simulink model "ORC_test_simu_feedback"  (R2018a)
settings: Solver=VariableStepAuto  StartTime=0.0  StopTime=9  RelTol=1e-4
undefined symbols (not defined in the file or in its folder): handle_sink, handle_source, handle_wf, pe, sigbuilder_block
libraries: pe_lib x1
(part 1 of 3)
settings Model: Creator=njgreen3  LastModifiedBy=njgreen3
settings SolverCC: AlgebraicLoopSolver=LineSearch
settings DebuggingCC: ParameterOverflowMsg=warning

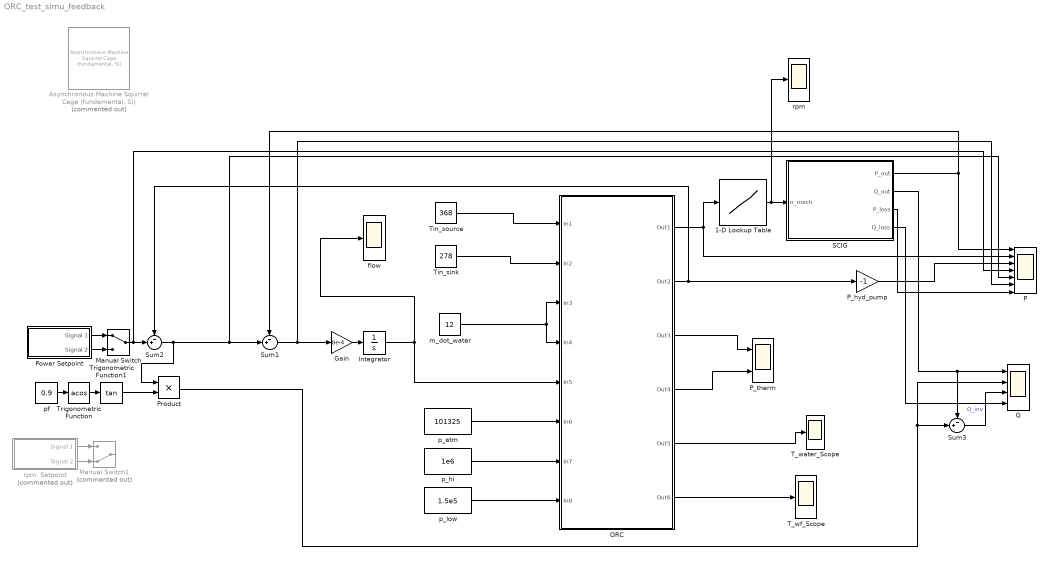
== system ORC_test_simu_feedback ==
  1-D Lookup Table : Lookup_n-D  NumberOfTableDimensions=1  BreakpointsForDimension1="-1/3*[166663.989372846\t163937.628261044\t155852.617467788\t140628.948970298\t116654.771019611\t83123.6124212207\t40806.0621676137\t-7481.19463142690\t-57239.4174183274\t-103560.341265182\t-142633.126036591\t-172599.754334336\t-193461.262910890\t-206409.980979167\t-213110.460435838\t-215209.127126632]"  Table="[834.591559026165\t844.140855611678\t853.690152197192\t863.239448782706\t872.788745368220\t882.338041953733\t891.887338539247\t901.436635124761\t910.985931710274\t920.535228295788\t930.084524881302\t939.633821466816\t949.183118052329\t958.732414637843\t968.281711223357\t977.831007808871]"  ExtrapMethod=Clip  DiagnosticForOutOfRangeInput=Error  InternalRulePriority=Speed  RndMeth=Simplest  InputSameDT=on
  "Asynchronous Machine Squirrel Cage (fundamental, SI)" : pe_lib/Machines/Asynchronous Machine (Squirrel Cage)/Asynchronous Machine Squirrel Cage (fundamental, SI)  Commented=on  SRated=40e3 V*A  VRated=220 V  FRated=60 Hz  nPolePairs=4  zero_sequence=pe.enum.park.zerosequence.include  Rs=0.018 Ohm  Xls=0.32 Ohm  Rrd=0.03 Ohm  Xlrd=0.05 Ohm  Xm=18 Ohm  X0=0.9 Ohm  connection_option=int32(pe.Connection.delta)  base_psi=nan Wb  angular_position_specify=off  angular_position_priority=None  angular_position=0 deg  angular_position_nominal_specify=off  angular_position_nominal_unit=deg  angular_position_nominal_value=1  psids_specify=off  psids_priority=None  psids=0 Wb  psids_nominal_specify=off  psids_nominal_unit=Wb  psids_nominal_value=1  psiqs_specify=off  psiqs_priority=None  psiqs=0 Wb  psiqs_nominal_specify=off  psiqs_nominal_unit=Wb  psiqs_nominal_value=1  psidr_specify=off  psidr_priority=None  psidr=0 Wb  psidr_nominal_specify=off  psidr_nominal_unit=Wb  psidr_nominal_value=1  psiqr_specify=off  psiqr_priority=None  psiqr=0 Wb  psiqr_nominal_specify=off  psiqr_nominal_unit=Wb  psiqr_nominal_value=1
      settings: SourceProductName=Simscape Power Systems  SourceProductBaseCode=PS
  Gain : Gain  Gain=8e-4
  Integrator : Integrator  InitialCondition=3  UpperSaturationLimit=8  LowerSaturationLimit=0
  Manual Switch : ManualSwitch
  Manual Switch1 : ManualSwitch  Commented=on  CurrentSetting=0
  ORC : Subsystem
  P : Scope  NumInputPorts=7
  P_hyd_pump : Gain  Gain=-1
  P_therm : Scope  NumInputPorts=2
  Power Setpoint : Subsystem  Tag=STV Subsys  LoadFcn=sigbuilder_block('load');  StartFcn=sigbuilder_block('start');  StopFcn=sigbuilder_block('stop');  ClipboardFcn=sigbuilder_block('clipboard');  mask(Sigbuilder block){tuvar=[0:10]}
      mask help: Simulink:masks:SigbuilderBlock_MD
      mask init:
      | if ~strcmp(get_param(bdroot(gcbh),'SimulationStatus'),'stopped') tuvar = sigbuilder_block('maskInit'); end
      settings: CopyFcn=sigbuilder_block('copy');  DeleteFcn=sigbuilder_block('delete');  ModelCloseFcn=sigbuilder_block('modelClose');  PreSaveFcn=sigbuilder_block('preSave');  PauseFcn=sigbuilder_block('pause');  ContinueFcn=sigbuilder_block('continue');  NameChangeFcn=sigbuilder_block('namechange');  OpenFcn=sigbuilder_block('open',[440.25 156.75 544.5 355.5 ]);  CloseFcn=sigbuilder_block('close');
      mask Display: plot(0, 0, 100, 100,[2, 2, 32, 32, 2], [68, 8, 8, 68, 68],[32, 2], [38, 38], [32, 19, 2],[53, 60, 44], [32, 17, 17, 2],[16, 16, 31, 31]);txt = getActiveGroup(gcbh);text(2, 100, txt,'verticalAlignment', 'top');
  Product : Product
  Q : Scope  NumInputPorts=4
  SCIG : MATLAB Function  TreatAsAtomicUnit=on  mask{Vll=220, f_synch=60, poles=4, R1=0.018, X1=0.32, R2=0.03, X2=0.05, Rm=5000, Xm=18, Rx=.003, Xx=12, K_b=0, K_w=0}
      mask prompts: Vll "Line Voltage (V)"; f_synch "Frequency (Hz)"; poles "Pole Pairs"; R1 "Stator Resistance, Rs"; X1 "Stator Reactance, Xs"; R2 "Referred Rotor Resistance, Rr'"; X2 "Reffered Rotor Reactance, Xr'"; Rm "Magnetizing Resistance of Core, Rm"; Xm "Magnetizing Reactance of Core, Xm"; Rx "Equivalent Series Resistance (ESR) of excitationm, Rx"; Xx "Excitation capacitance, Xx"; K_b "Coefficient of Bearing Friction, Kb"; K_w "Coefficient of Windage Friction, Kw"
  Sum1 : Sum  Inputs=-+|
  Sum2 : Sum  Inputs=-+|
  Sum3 : Sum  Inputs=-+|
  T_water_Scope : Scope
  T_wf_Scope : Scope
  Tin_sink : Constant  Value=278
  Tin_source : Constant  Value=368
  Trigonometric Function : Trigonometry  Operator=acos
  Trigonometric Function1 : Trigonometry  Operator=tan
  flow : Scope
  m_dot_water : Constant  Value=12
  p_atm : Constant  Value=101325
  p_hi : Constant  Value=1e6
  p_low : Constant  Value=1.5e5
  pf : Constant  Value=0.9
  rpm : Scope
  rpm  Setpoint : Subsystem  Tag=STV Subsys  Commented=on  LoadFcn=sigbuilder_block('load');  StartFcn=sigbuilder_block('start');  StopFcn=sigbuilder_block('stop');  ClipboardFcn=sigbuilder_block('clipboard');  mask(Sigbuilder block){tuvar=[0:10]}
      mask help: Simulink:masks:SigbuilderBlock_MD
      mask init:
      | if ~strcmp(get_param(bdroot(gcbh),'SimulationStatus'),'stopped') tuvar = sigbuilder_block('maskInit'); end
      settings: CopyFcn=sigbuilder_block('copy');  DeleteFcn=sigbuilder_block('delete');  ModelCloseFcn=sigbuilder_block('modelClose');  PreSaveFcn=sigbuilder_block('preSave');  PauseFcn=sigbuilder_block('pause');  ContinueFcn=sigbuilder_block('continue');  NameChangeFcn=sigbuilder_block('namechange');  OpenFcn=sigbuilder_block('open',[674.25 225 550.5 399.75 ]);  CloseFcn=sigbuilder_block('close');
      mask Display: plot(0, 0, 100, 100,[2, 2, 32, 32, 2], [68, 8, 8, 68, 68],[32, 2], [38, 38], [32, 19, 2],[53, 60, 44], [32, 17, 17, 2],[16, 16, 31, 31]);txt = getActiveGroup(gcbh);text(2, 100, txt,'verticalAlignment', 'top');
  wires:
  Tin_source/1 -> ORC/1(In1)
  m_dot_water/1 -> ORC/3(In3), ORC/4(In4)
  p_atm/1 -> ORC/6(In6)
  p_hi/1 -> ORC/7(In7)
  p_low/1 -> ORC/8(In8)
  ORC/3(Out3) -> P_therm/1
  ORC/4(Out4) -> P_therm/2
  ORC/5(Out5) -> T_water_Scope/1
  ORC/6(Out6) -> T_wf_Scope/1
  Tin_sink/1 -> ORC/2(In2)
  Gain/1 -> Integrator/1
  Power Setpoint/1(Signal 1) -> Manual Switch/1
  Power Setpoint/2(Signal 2) -> Manual Switch/2
  Manual Switch/1 -> P/4, Sum2/2
  pf/1 -> Trigonometric Function/1
  Trigonometric Function/1 -> Trigonometric Function1/1
  Trigonometric Function1/1 -> Product/2
  Product/1 -> Sum3/2, Q/2
  Sum2/1 -> P/5, Sum1/2, Product/1
  rpm  Setpoint/1(Signal 1) -> Manual Switch1/1
  rpm  Setpoint/2(Signal 2) -> Manual Switch1/2
  Integrator/1 -> ORC/5(In5), flow/1
  ORC/1(Out1) -> P/2, 1-D Lookup Table/1
  1-D Lookup Table/1 -> rpm/1, SCIG/1(n_mech)
  ORC/2(Out2) -> Sum2/1, P_hyd_pump/1
  SCIG/1(P_out) -> Sum1/1, P/1
  P_hyd_pump/1 -> P/3
  Sum1/1 -> P/6, Gain/1
  SCIG/2(Q_out) -> Sum3/1, Q/1
  Sum3/1 -> Q/3  "Q_inv"
  SCIG/4(Q_loss) -> Q/4
  SCIG/3(P_loss) -> P/7

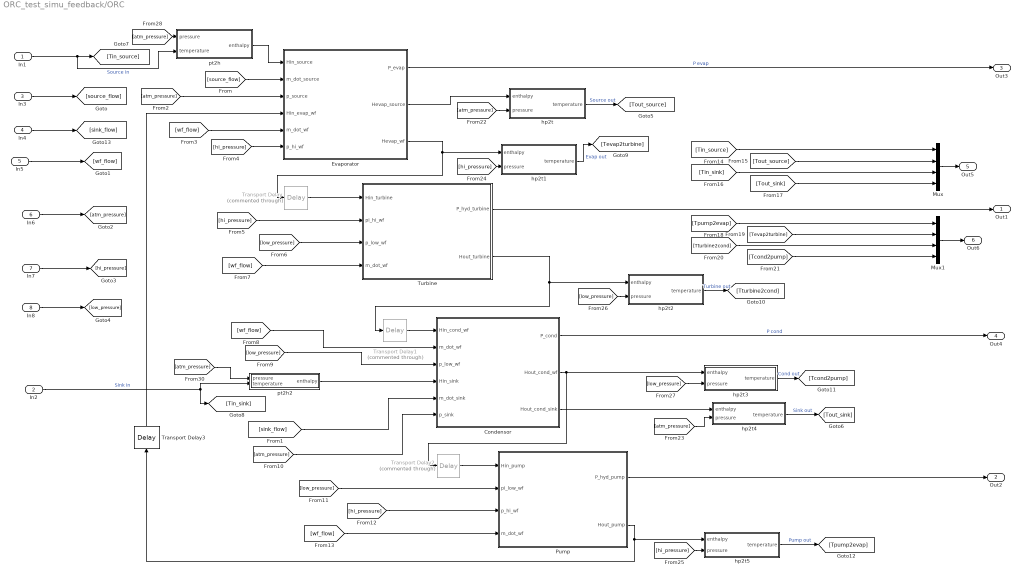
== system ORC_test_simu_feedback/ORC ==
  In1 : Inport
  In2 : Inport  Port=2
  In3 : Inport  Port=3
  In4 : Inport  Port=4
  In5 : Inport  Port=5
  In6 : Inport  Port=6
  In7 : Inport  Port=7
  In8 : Inport  Port=8
  Condensor : Subsystem
  Evaporator : Subsystem
  Mux : Mux
  Mux1 : Mux
  Pump : Subsystem
  Transport Delay : TransportDelay  Commented=through  DelayTime=.01  InitialOutput=2.3e+05
  Transport Delay1 : TransportDelay  Commented=through  DelayTime=.01  InitialOutput=2.3e+05
  Transport Delay2 : TransportDelay  Commented=through  DelayTime=.01  InitialOutput=2.3e+05
  Transport Delay3 : TransportDelay  DelayTime=.01  InitialOutput=2.3e+05  TransDelayFeedthrough=on
  Turbine : Subsystem
  hp2t : MATLAB Function  TreatAsAtomicUnit=on  mask{fluid_handle=handle_source}
      mask prompts: fluid_handle "Fluid Handle"
  hp2t1 : MATLAB Function  TreatAsAtomicUnit=on  mask{fluid_handle=handle_wf}
      mask prompts: fluid_handle "Fluid Handle"
  hp2t2 : MATLAB Function  TreatAsAtomicUnit=on  mask{fluid_handle=handle_wf}
      mask prompts: fluid_handle "Fluid Handle"
  hp2t3 : MATLAB Function  TreatAsAtomicUnit=on  mask{fluid_handle=handle_wf}
      mask prompts: fluid_handle "Fluid Handle"
  hp2t4 : MATLAB Function  TreatAsAtomicUnit=on  mask{fluid_handle=handle_sink}
      mask prompts: fluid_handle "Fluid Handle"
  hp2t5 : MATLAB Function  TreatAsAtomicUnit=on  mask{fluid_handle=handle_wf}
      mask prompts: fluid_handle "Fluid Handle"
  pt2h : MATLAB Function  TreatAsAtomicUnit=on  mask{fluid_handle=handle_source}
      mask prompts: fluid_handle "Fluid Handle"
  pt2h2 : MATLAB Function  TreatAsAtomicUnit=on  mask{fluid_handle=handle_sink}
      mask prompts: fluid_handle "Fluid Handle"
  Out1 : Outport
  Out2 : Outport  Port=2
  Out3 : Outport  Port=3
  Out4 : Outport  Port=4
  Out5 : Outport  Port=5
  Out6 : Outport  Port=6
  wires:
  [wf_flow] -> Pump/4(m_dot_wf)
  Pump/2(Hout_pump) -> Transport Delay3/1, hp2t5/1(enthalpy)
  [Tturbine2cond] -> Mux1/3
  Condensor/2(Hout_cond_wf) -> hp2t3/1(enthalpy), Transport Delay2/1
  Transport Delay1/1 -> Condensor/1(Hin_cond_wf)
  In3/1 -> [source_flow]
  Transport Delay3/1 -> Evaporator/4(Hin_evap_wf)
  [atm_pressure] -> Evaporator/3(p_source)
  Evaporator/3(Hevap_wf) -> Transport Delay/1, hp2t1/1(enthalpy)
  Transport Delay/1 -> Turbine/1(Hin_turbine)
  In1/1 -> pt2h/2(temperature), [Tin_source]  "Source in"
  hp2t2/1(temperature) -> [Tturbine2cond]  "Turbine out"
  [atm_pressure] -> hp2t4/2(pressure)
  [wf_flow] -> Evaporator/5(m_dot_wf)
  [hi_pressure] -> Pump/3(p_hi_wf)
  Turbine/2(Hout_turbine) -> Transport Delay1/1, hp2t2/1(enthalpy)
  [low_pressure] -> Condensor/3(p_low_wf)
  [hi_pressure] -> Evaporator/6(p_hi_wf)
  [low_pressure] -> Turbine/3(p_low_wf)
  [wf_flow] -> Turbine/4(m_dot_wf)
  [wf_flow] -> Condensor/2(m_dot_wf)
  [Tcond2pump] -> Mux1/4
  [sink_flow] -> Condensor/5(m_dot_sink)
  [atm_pressure] -> Condensor/6(p_sink)
  Evaporator/2(Hevap_source) -> hp2t/1(enthalpy)
  [low_pressure] -> hp2t3/2(pressure)
  [hi_pressure] -> Turbine/2(pi_hi_wf)
  [atm_pressure] -> pt2h/1(pressure)
  Transport Delay2/1 -> Pump/1(Hin_pump)
  hp2t4/1(temperature) -> [Tout_sink]  "Sink out"
  hp2t/1(temperature) -> [Tout_source]  "Source out"
  [low_pressure] -> Pump/2(pi_low_wf)
  hp2t1/1(temperature) -> [Tevap2turbine]  "Evap out"
  hp2t3/1(temperature) -> [Tcond2pump]  "Cond out"
  hp2t5/1(temperature) -> [Tpump2evap]  "Pump out"
  [low_pressure] -> hp2t2/2(pressure)
  [hi_pressure] -> hp2t5/2(pressure)
  [source_flow] -> Evaporator/2(m_dot_source)
  [atm_pressure] -> pt2h2/1(pressure)
  [hi_pressure] -> hp2t1/2(pressure)
  [atm_pressure] -> hp2t/2(pressure)
  pt2h2/1(enthalpy) -> Condensor/4(Hin_sink)
  Condensor/3(Hout_cond_sink) -> hp2t4/1(enthalpy)
  pt2h/1(enthalpy) -> Evaporator/1(Hin_source)
  In2/1 -> pt2h2/2(temperature), [Tin_sink]  "Sink in"
  [Tout_source] -> Mux/2
  In7/1 -> [hi_pressure]
  In5/1 -> [wf_flow]
  In8/1 -> [low_pressure]
  In6/1 -> [atm_pressure]
  [Tin_source] -> Mux/1
  [Tin_sink] -> Mux/3
  [Tevap2turbine] -> Mux1/2
  Evaporator/1(P_evap) -> Out3/1  "P evap"
  Pump/1(P_hyd_pump) -> Out2/1
  Condensor/1(P_cond) -> Out4/1  "P cond"
  [Tpump2evap] -> Mux1/1
  Turbine/1(P_hyd_turbine) -> Out1/1
  [Tout_sink] -> Mux/4
  Mux/1 -> Out5/1
  Mux1/1 -> Out6/1
  In4/1 -> [sink_flow]

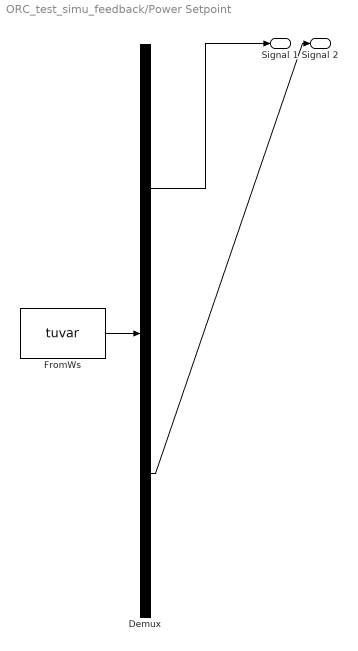
== system ORC_test_simu_feedback/Power Setpoint ==
  Demux : Demux  Tag=STV Demux  Outputs=2
  FromWs : FromWorkspace  Tag=STV FromWs  VariableName=tuvar  SampleTime=0
      SigBuilderData=|
      | common.afterFinalStr = 'Extrapolate'
      | common.sampleTime = 0
      | dataSet.timeRange = [0 8]
      | dataSet.name = 'Group 1'
      | sbobj.Groups.Name = 'Group 1'
      | sbobj.Groups.Signals(1).Name = 'Signal 1'
      | sbobj.Groups.Signals(1).XData = [0 1.5 1.5 3 3 4.5 4.5 7.02 7.02 8]
      | sbobj.Groups.Signals(1).YData = [15000 15000 20200 20200 25000 25000 30000 30000 25600 25600]
      | sbobj.Groups.Signals(2).Name = 'Signal 2'
      | sbobj.Groups.Signals(2).XData = [0 8]
      | sbobj.Groups.Signals(2).YData = [20000 20000]
      | sbobj.Groups.TimeRange = [0 8]
  Signal 1 : Outport  Tag=STV Outport
  Signal 2 : Outport  Tag=STV Outport  Port=2
  wires:
  Demux/1 -> Signal 1/1
  FromWs/1 -> Demux/1
  Demux/2 -> Signal 2/1

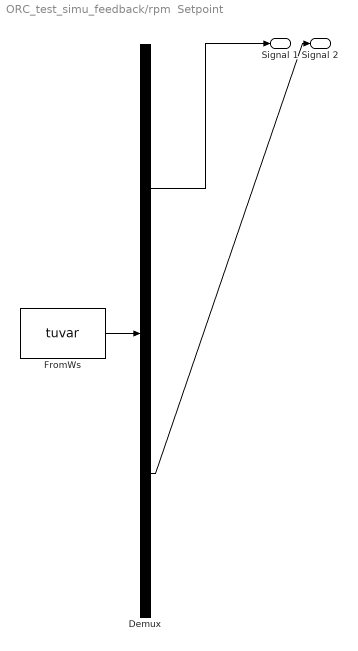
== system ORC_test_simu_feedback/rpm  Setpoint ==
  Demux : Demux  Tag=STV Demux  Outputs=2
  FromWs : FromWorkspace  Tag=STV FromWs  VariableName=tuvar  SampleTime=0
      SigBuilderData=|
      | common.afterFinalStr = 'Extrapolate'
      | common.sampleTime = 0
      | dataSet.timeRange = [0 10]
      | dataSet.name = 'Group 1'
      | sbobj.Groups.Name = 'Group 1'
      | sbobj.Groups.Signals(1).Name = 'Signal 1'
      | sbobj.Groups.Signals(1).XData = [0 4 6 6 9.1 9.1 9.38 9.38 10]
      | sbobj.Groups.Signals(1).YData = [904 904 948 950 952 914 916 915 915]
      | sbobj.Groups.Signals(2).Name = 'Signal 2'
      | sbobj.Groups.Signals(2).XData = [0 10]
      | sbobj.Groups.Signals(2).YData = [911 911]
  Signal 1 : Outport  Tag=STV Outport
  Signal 2 : Outport  Tag=STV Outport  Port=2
  wires:
  Demux/1 -> Signal 1/1
  FromWs/1 -> Demux/1
  Demux/2 -> Signal 2/1

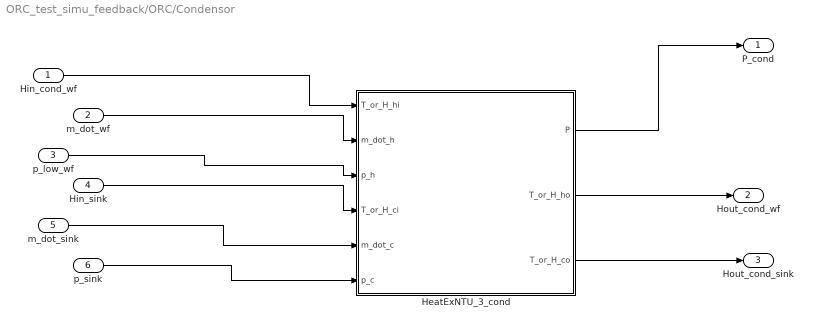
== system ORC_test_simu_feedback/ORC/Condensor ==
  Hin_cond_wf : Inport
  m_dot_wf : Inport  Port=2
  p_low_wf : Inport  Port=3
  Hin_sink : Inport  Port=4
  m_dot_sink : Inport  Port=5
  p_sink : Inport  Port=6
  HeatExNTU_3_cond : MATLAB Function  Description=|  TreatAsAtomicUnit=on  mask{U=1400, A=18.6, HeatExType=counter, fluid_h=handle_wf, fluid_c=handle_sink, T_or_H=0}
      | %HeatExNTU Summary 
      | %   This function calculates flow and outlet temperatures of a heat exchanger
      | %   using the Number of Transfer Units (NTU) method as described in
      | %   Fundementals of Heat and Mass Transfer by F. P. Incropera, D. P.
      | %   DeWitt, T. L. Bergman & A. S. Lavine. The method can be used when only
      | %   the inlet tempertures are known as opposed to inlet and outlet
      | %   temperatures.
      | %
      | %   This is done by calculating effectiveness which is defined as the ratio
      | %   of actual heat transferred to the maximum possible heat transferred for 
      | %   an infinite length counter-flow heat exchanger with the given inlet
      | %   temperatures. The effectivenes is calculated differently depending on 
      | %   the geometry of exchanger but is always a function of the ratio of heat
      | %   capacity rates as well as the number of transfer units (NTU). The NTU
      | %   depends on the overall heat transfer coefficient, the heat transfer
      | %   area, and the smaller of the two heat capacity rates. 
      | %   
      | %   In the event of a phase change the rate of change of energy required to
      | %   get the fluid just beyond the point of vaporizaion or condensation is
      | %   calculated using the CoolProp function. Then the function is called
      | %   again at the new temperature and the final temperatures and heat rates
      | %   are calucluated using a reduced heat exhange area. I currently assume
      | %   the effected heat transfer area is a half of the original input. This 
      | %   function cannot accurately handle both fluids changing phase because it
      | %   does not check which fluid would change first.
      | % 
      | % Note: The effectiveness is separte from efficiency. The calculations
      | %   assumes an efficiency of 1 where all heat is transferred from the hot
      | %   fluid to the cool fluid or remains within the the fluid. This also
      | %   assumes no fluid is undergoing a change in state, which may not be
      | %   sufficient for my final model.
      | %
      | % This function makes use of the CoolProp wrapper for fluid properties. 
      | % The high level Matlab wrapper cannot handle vector inputs. There ways to
      | % make low level calls interfacing with the DLL so many values can be
      | % determined more quickly, but that is not implented here.
      | % More information about the Matlab wrapper can be found at
      | %   http://www.coolprop.org/coolprop/wrappers/MATLAB/index.html
      | % A list of parameters can be found at 
      | %   http://www.coolprop.org/coolprop/HighLevelAPI.html#parameter-table
      | % A list of fluids can be found at 
      | %   http://www.coolprop.org/fluid_properties/PurePseudoPure.html#list-of-fluids
      | %
      | % Inputs:
      | %   Thi         Hot fluid inlet temperature in Kelvin
      | %   m_dot_h     Hot fluid mass flow rate in kg/s
      | %   p_h         Hot fluid pressure in pa
      | %   fluid_h     Name of Hot fluid (string)
      | %   Tci         Cool fluid inlet temperature in Kelvin
      | %   m_dot_c     Cool fluid mass flow rate in kg/s
      | %   p_c         Cool fluid pressure in pa
      | %   fluid_c     Name of Cool fluid (string)
      | %   HeatExType  String describing the heat exchanger geometry. Currently
      | %               this variable only accepts 'counter' and 'parallel', but
      | %               can be expanded to other exchanger/flow types
      | %               'counter' for counter flow
      | %               'parallel' for parallel
      | %   U           Overall heat transfer coefficient in W/(K m2)
      | %   A           Heat transfer area in m2
      | %
      | % Output:
      | %   P           Rate of heat exchenged (power) in W
      | %   Tho         Hot fluid outlet temperature in input temp units (K)
      | %   Tco         Cool fluid outlet temperature in input tempt units (K)
      mask prompts: U "Heat Transfer Coefficient"; A "Heat Transfer Area"; HeatExType "Heat Exchanger Type"; fluid_h "Hot Fluid Handle"; fluid_c "Cool Fluid Handle"; T_or_H "Temperature(1) or Enthalpy(0)"
  P_cond : Outport
  Hout_cond_wf : Outport  Port=2
  Hout_cond_sink : Outport  Port=3
  wires:
  Hin_cond_wf/1 -> HeatExNTU_3_cond/1(T_or_H_hi)
  m_dot_wf/1 -> HeatExNTU_3_cond/2(m_dot_h)
  p_low_wf/1 -> HeatExNTU_3_cond/3(p_h)
  p_sink/1 -> HeatExNTU_3_cond/6(p_c)
  m_dot_sink/1 -> HeatExNTU_3_cond/5(m_dot_c)
  Hin_sink/1 -> HeatExNTU_3_cond/4(T_or_H_ci)
  HeatExNTU_3_cond/1(P) -> P_cond/1
  HeatExNTU_3_cond/2(T_or_H_ho) -> Hout_cond_wf/1
  HeatExNTU_3_cond/3(T_or_H_co) -> Hout_cond_sink/1

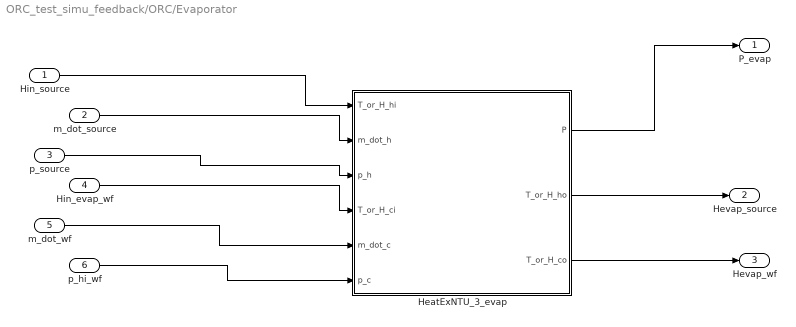
== system ORC_test_simu_feedback/ORC/Evaporator ==
  Hin_source : Inport
  m_dot_source : Inport  Port=2
  p_source : Inport  Port=3
  Hin_evap_wf : Inport  Port=4
  m_dot_wf : Inport  Port=5
  p_hi_wf : Inport  Port=6
  HeatExNTU_3_evap : MATLAB Function  Description=|  TreatAsAtomicUnit=on  mask{U=1500, A=9.3, HeatExType=counter, fluid_h=handle_source, fluid_c=handle_wf, T_or_H=0}
      | %HeatExNTU Summary 
      | %   This function calculates flow and outlet temperatures of a heat exchanger
      | %   using the Number of Transfer Units (NTU) method as described in
      | %   Fundementals of Heat and Mass Transfer by F. P. Incropera, D. P.
      | %   DeWitt, T. L. Bergman & A. S. Lavine. The method can be used when only
      | %   the inlet tempertures are known as opposed to inlet and outlet
      | %   temperatures.
      | %
      | %   This is done by calculating effectiveness which is defined as the ratio
      | %   of actual heat transferred to the maximum possible heat transferred for 
      | %   an infinite length counter-flow heat exchanger with the given inlet
      | %   temperatures. The effectivenes is calculated differently depending on 
      | %   the geometry of exchanger but is always a function of the ratio of heat
      | %   capacity rates as well as the number of transfer units (NTU). The NTU
      | %   depends on the overall heat transfer coefficient, the heat transfer
      | %   area, and the smaller of the two heat capacity rates. 
      | %   
      | %   In the event of a phase change the rate of change of energy required to
      | %   get the fluid just beyond the point of vaporizaion or condensation is
      | %   calculated using the CoolProp function. Then the function is called
      | %   again at the new temperature and the final temperatures and heat rates
      | %   are calucluated using a reduced heat exhange area. I currently assume
      | %   the effected heat transfer area is a half of the original input. This 
      | %   function cannot accurately handle both fluids changing phase because it
      | %   does not check which fluid would change first.
      | % 
      | % Note: The effectiveness is separte from efficiency. The calculations
      | %   assumes an efficiency of 1 where all heat is transferred from the hot
      | %   fluid to the cool fluid or remains within the the fluid. This also
      | %   assumes no fluid is undergoing a change in state, which may not be
      | %   sufficient for my final model.
      | %
      | % This function makes use of the CoolProp wrapper for fluid properties. 
      | % The high level Matlab wrapper cannot handle vector inputs. There ways to
      | % make low level calls interfacing with the DLL so many values can be
      | % determined more quickly, but that is not implented here.
      | % More information about the Matlab wrapper can be found at
      | %   http://www.coolprop.org/coolprop/wrappers/MATLAB/index.html
      | % A list of parameters can be found at 
      | %   http://www.coolprop.org/coolprop/HighLevelAPI.html#parameter-table
      | % A list of fluids can be found at 
      | %   http://www.coolprop.org/fluid_properties/PurePseudoPure.html#list-of-fluids
      | %
      | % Inputs:
      | %   Thi         Hot fluid inlet temperature in Kelvin
      | %   m_dot_h     Hot fluid mass flow rate in kg/s
      | %   p_h         Hot fluid pressure in pa
      | %   fluid_h     Name of Hot fluid (string)
      | %   Tci         Cool fluid inlet temperature in Kelvin
      | %   m_dot_c     Cool fluid mass flow rate in kg/s
      | %   p_c         Cool fluid pressure in pa
      | %   fluid_c     Name of Cool fluid (string)
      | %   HeatExType  String describing the heat exchanger geometry. Currently
      | %               this variable only accepts 'counter' and 'parallel', but
      | %               can be expanded to other exchanger/flow types
      | %               'counter' for counter flow
      | %               'parallel' for parallel
      | %   U           Overall heat transfer coefficient in W/(K m2)
      | %   A           Heat transfer area in m2
      | %
      | % Output:
      | %   P           Rate of heat exchenged (power) in W
      | %   Tho         Hot fluid outlet temperature in input temp units (K)
      | %   Tco         Cool fluid outlet temperature in input tempt units (K)
      mask prompts: U "Heat Transfer Coefficient"; A "Heat Transfer Area"; HeatExType "Heat Exchanger Type"; fluid_h "Hot Fluid Handle"; fluid_c "Cool Fluid Handle"; T_or_H "Temperature (1) or Enthalpy (0)"
      mask init:
      | % set_param('ORC_test_simu/Evaporator/HeatExNTU_3_block', 'fluid_h', 'Water')
  P_evap : Outport
  Hevap_source : Outport  Port=2
  Hevap_wf : Outport  Port=3
  wires:
  Hin_source/1 -> HeatExNTU_3_evap/1(T_or_H_hi)
  m_dot_source/1 -> HeatExNTU_3_evap/2(m_dot_h)
  p_source/1 -> HeatExNTU_3_evap/3(p_h)
  p_hi_wf/1 -> HeatExNTU_3_evap/6(p_c)
  m_dot_wf/1 -> HeatExNTU_3_evap/5(m_dot_c)
  Hin_evap_wf/1 -> HeatExNTU_3_evap/4(T_or_H_ci)
  HeatExNTU_3_evap/1(P) -> P_evap/1
  HeatExNTU_3_evap/2(T_or_H_ho) -> Hevap_source/1
  HeatExNTU_3_evap/3(T_or_H_co) -> Hevap_wf/1

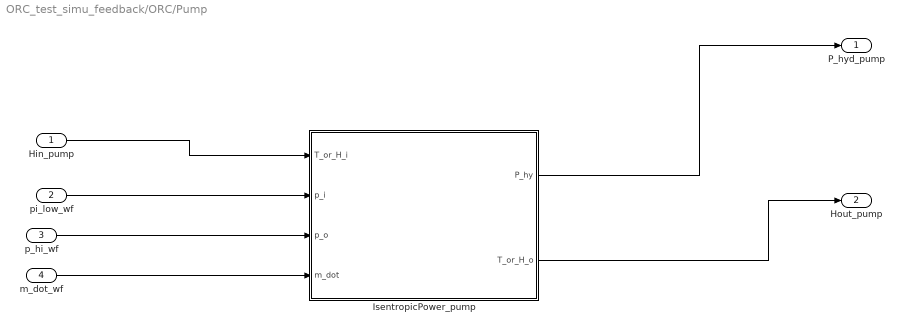
== system ORC_test_simu_feedback/ORC/Pump ==
  Hin_pump : Inport
  pi_low_wf : Inport  Port=2
  p_hi_wf : Inport  Port=3
  m_dot_wf : Inport  Port=4
  IsentropicPower_pump : MATLAB Function  TreatAsAtomicUnit=on  mask{isen_eff=.78, T_or_H=0, fluid=handle_wf}
      mask prompts: isen_eff "Isentropic Efficiency"; T_or_H "Temperature (1) or Enthalpy (0)"; fluid "Fluid Handle"
  P_hyd_pump : Outport
  Hout_pump : Outport  Port=2
  wires:
  pi_low_wf/1 -> IsentropicPower_pump/2(p_i)
  m_dot_wf/1 -> IsentropicPower_pump/4(m_dot)
  Hin_pump/1 -> IsentropicPower_pump/1(T_or_H_i)
  IsentropicPower_pump/1(P_hy) -> P_hyd_pump/1
  IsentropicPower_pump/2(T_or_H_o) -> Hout_pump/1
  p_hi_wf/1 -> IsentropicPower_pump/3(p_o)

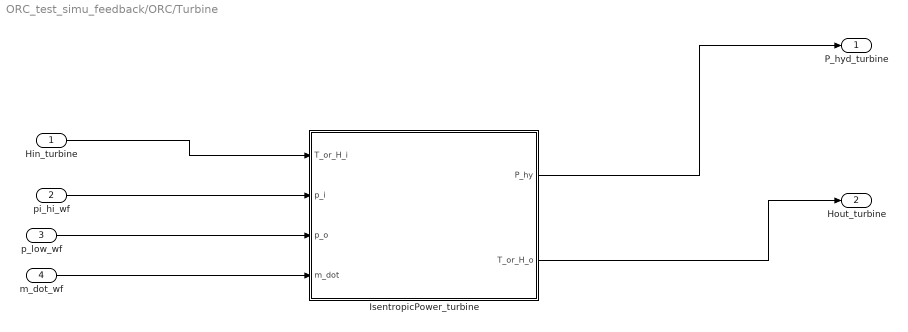
== system ORC_test_simu_feedback/ORC/Turbine ==
  Hin_turbine : Inport
  pi_hi_wf : Inport  Port=2
  p_low_wf : Inport  Port=3
  m_dot_wf : Inport  Port=4
  IsentropicPower_turbine : MATLAB Function  TreatAsAtomicUnit=on  mask{isen_eff=.78, T_or_H=0, fluid=handle_wf}
      mask prompts: isen_eff "Isentropic Efficiency"; T_or_H "Temperature (1) or Enthalpy (0)"; fluid "Fluid Handle"
  P_hyd_turbine : Outport
  Hout_turbine : Outport  Port=2
  wires:
  pi_hi_wf/1 -> IsentropicPower_turbine/2(p_i)
  m_dot_wf/1 -> IsentropicPower_turbine/4(m_dot)
  Hin_turbine/1 -> IsentropicPower_turbine/1(T_or_H_i)
  IsentropicPower_turbine/1(P_hy) -> P_hyd_turbine/1
  IsentropicPower_turbine/2(T_or_H_o) -> Hout_turbine/1
  p_low_wf/1 -> IsentropicPower_turbine/3(p_o)

== matlab function ORC_test_simu_feedback/ORC/Turbine/IsentropicPower_turbine ==
  data: T_or_H_i input; P_hy output; p_i input; p_o input; m_dot input; T_or_H_o output; T_or_H parameter; isen_eff parameter; fluid parameter
function [ P_hy, T_or_H_o ] = IsentropicPower_block( T_or_H_i, p_i, p_o, m_dot, T_or_H,  isen_eff, fluid)
% function [ P_hy ] = IsentropicPower( T_i, T_o, p_i, p_o, m_dot, fluid, isen_eff )
%EXPANDER Summary of this function
%   This process calculates the mechanical power provided or required by a 
%   generic expander device/system. Turbines and other expanders provide
%   mechanical power while pumps and compressors consume it. This is done
%   by calculating the change in enthalpy of fluid and multipying by the 
%   mass flow rate while entropy remains constant.  Non ideal processes are
%   taken into account through the isentropic efficiency.
% 
% Inputs:
%   T_or_H_i    Input temperature in Kelvin or enthalpy in J/kg
%   p_i         Input pressure of the fluid in Pa
%   p_o         Output temperature of the fluid in Pa
%   m_dot       Mass flow rate of the fluid in kg/s 
%   fluid       Initialzed coolprop fluid handle
%   isen_eff    Isentropic efficiency of the device. Expected range: 0-1
%               This input is optional. If it is not provided then it will 
%               be set to 1, which is the efficiency of an ideal isentropic
%               device where entropy is constant.
%               This value is treated differently depending on if there is
%               an increase or decrease in fluid enthalpy. If the enthalpy
%               decreases (energy is extracted from the system) then the
%               efficiency if multiplied by the change in energy because
%               less energy is extracted than the ideal case. If the
%               enthalpy increases (energy in added to the system) then the
%               efficiency is divided by the change in energy because more
%               energy is required than the ideal case.
%   T_or_H      Logical indicating whether the relavent input and output
%               variables are temperature (1) or enthalpy (0)
% 
% Outputs:
%   P_hy        Hydraulic power exctracted or consumed in W. Positive
%               values indicate the system is providing hydraulic power as
%               a turbine or expander. Negative values indicate the system 
%               is consuming hydraulic power as a compressor or pump.
%   T_or_H_o    Output temperature in Kelvin or enthalpy in J/kg

% This function makes use of the CoolProp wrapper for fluid properties. 
% The high level Matlab wrapper cannot handle vector inputs. There ways to
% make low level calls interfacing with the DLL so many values can be
% determined more quickly, but that is not implented here.
% More information about the Matlab wrapper can be found at
%   http://www.coolprop.org/coolprop/wrappers/MATLAB/index.html
% A list of parameters can be found at 
%   http://www.coolprop.org/coolprop/HighLevelAPI.html#parameter-table
% A list of fluids can be found at 
%   http://www.coolprop.org/fluid_properties/PurePseudoPure.html#list-of-fluids

% initailize certain parameters used to call coolprop library
buffer_size = 255;
ierr = 0;
b = (1:1:buffer_size);
herr= char(b);
coder.extrinsic('calllib') 
coder.extrinsic('libpointer') 

% All the input signals should be the same size, so it shouldn't matter
% which one is used to obtain signal length
var_length = length(T_or_H_i);

% determine input parameter pair indecies for coolprop calls
% [pq_ind,~] = calllib('coolprop','get_input_pair_index','PQ_INPUTS'); %pressure and Mass vapor quality
[pt_ind,~] = calllib('coolprop','get_input_pair_index','PT_INPUTS'); %pressure and temperature
[hp_ind,~] = calllib('coolprop','get_input_pair_index','HmassP_INPUTS'); %Mass specific enthalpy and pressure
[ps_ind,~] = calllib('coolprop','get_input_pair_index','PSmass_INPUTS'); %pressure and Mass specific entropy

% determine output parameter indecies for coolprop calls
[t_ind, ~] = calllib('coolprop','get_param_index','T'); %temperature
[s_ind, ~] = calllib('coolprop','get_param_index','S'); %Mass specific entropy
[h_ind, ~] = calllib('coolprop','get_param_index','Hmass'); %Mass specific enthalpy
% [c_ind, ~] = calllib('coolprop','get_param_index','Cpmass'); %Mass specific constant pressure specific heat

% find pointer location of pressure input and output values
p_i_Ptr = libpointer('doublePtr',p_i);
p_o_Ptr = libpointer('doublePtr',p_o);

% Ensure temperature/enthalpy input variables are delt with appropriately
if T_or_H 
% Assume given temperature values are not at vaporization/condensation.
% Initialize T and H inputs
    T_i = T_or_H_i;
    T_i_Ptr = libpointer('doublePtr',T_i);
    H_i = zeros(var_length,1); % initialized to 0 temporarily
    H_i_Ptr = libpointer('doublePtr',H_i);
% Update values located at Hhi and Hci pointer locations
    calllib('coolprop','AbstractState_update_and_1_out', fluid, pt_ind, p_i_Ptr, T_i_Ptr, var_length, h_ind, H_i_Ptr, ierr,herr,buffer_size);
% Set Hhi & Hci to values stored at pointer location
    H_i = get(H_i_Ptr,'Value');
    
else
% Enthalpy values can be in vaporization/condensation region  
% Initialize H values
    H_i = T_or_H_i;
    H_i_Ptr = libpointer('doublePtr',H_i);

end

% Input entropy in J/kg/K
% Initialize pointer locations for relevant variables
S_i_Ptr = libpointer('doublePtr', zeros(var_length,1)); 
% Update values at S_i pointer location
calllib('coolprop','AbstractState_update_and_1_out', fluid, hp_ind, H_i_Ptr, p_i_Ptr, var_length, s_ind, S_i_Ptr, ierr,herr,buffer_size);
% Set S_i to values stored at pointer location
% S_i = get(S_i_Ptr,'Value');

% Ideal Output entropy is equal to input entropy 
% Ideal Output enthalpy in J/kg and temperature
H_o_ideal = zeros(var_length,1);
H_o_ideal_Ptr = libpointer('doublePtr',H_o_ideal);
% Update values located at Hhi and Hci pointer locations
calllib('coolprop','AbstractState_update_and_1_out', fluid, ps_ind, p_o_Ptr, S_i_Ptr, var_length, h_ind, H_o_ideal_Ptr, ierr,herr,buffer_size);
% Set H_o_ideal to values stored at pointer location
H_o_ideal = get(H_o_ideal_Ptr,'Value');

% Calculate Ideal power consumed/provided
P_ideal = m_dot.*(H_i - H_o_ideal);

% Initialize hydrolic power variable
P_hy = zeros(var_length,1);
%   If positive then the system is providing power as a turbine
%   or expander.
%   This means the actual power provided is less than the ideal power
P_hy(P_ideal > 0) = isen_eff.*P_ideal(P_ideal > 0);

%   If negative then the system is consuming power as a
%   compressor or pump.
%   This means the actual power consumed is greater than the ideal power.
P_hy(P_ideal < 0) = P_ideal(P_ideal < 0)./isen_eff;

% Set output enthalpy
H_o = H_i - P_hy./m_dot;
H_o_Ptr = libpointer('doublePtr',H_o);

% Ensure temperature/enthalpy input variables are delt with appropriately
if T_or_H 
% Assume given temperature values are not at vaporization/condensation
    T_or_H_o = zeros(var_length,1);
    T_or_H_o_Ptr = libpointer('doublePtr',T_or_H_o);
    calllib('coolprop','AbstractState_update_and_1_out', fluid, hp_ind, H_o_Ptr, p_o_Ptr, var_length, t_ind, T_or_H_o_Ptr, ierr,herr,buffer_size);
    T_or_H_o = get(T_or_H_o_Ptr,'Value');
    
else
% Enthalpy values can be in vaporization/condensation region    
    T_or_H_o = H_o;
end
end
